simulink model "R1_double"  (R2014b)
settings: Solver=ode3  SolverMode=SingleTasking  StartTime=0.0  StopTime=Tsim  FixedStep=Ts  RelTol=1e-3
InitFcn:
  | configDoubleIntegrator
libraries: simulink x1
settings Model: CovMetricSettings=dwe  CovHtmlReporting=off  covSaveCumulativeToWorkspaceVar=off  CovSaveSingleToWorkspaceVar=off  CovExternalEMLEnable=on  CovSFcnEnable=on  Creator=mnade  LastModifiedBy=nina
settings DataIOCC: LimitDataPoints=off  SaveFormat=StructureWithTime
settings DebuggingCC: SolverPrmCheckMsg=none  FrameProcessingCompatibilityMsg=error  SFUnexpectedBacktrackingDiag=error  SFNoUnconditionalDefaultTransitionDiag=error
settings HardwareCC: ProdBitPerPointer=64  ProdLargestAtomicFloat=Float  ProdIntDivRoundTo=Zero  ProdEndianess=LittleEndian  ProdHWDeviceType=Specified
settings ModelReferenceCC: PropagateSignalLabelsOutOfModel=on
settings GRTTargetCC: TargetLangStandard=C99 (ISO)  GeneratePreprocessorConditionals=Use local settings

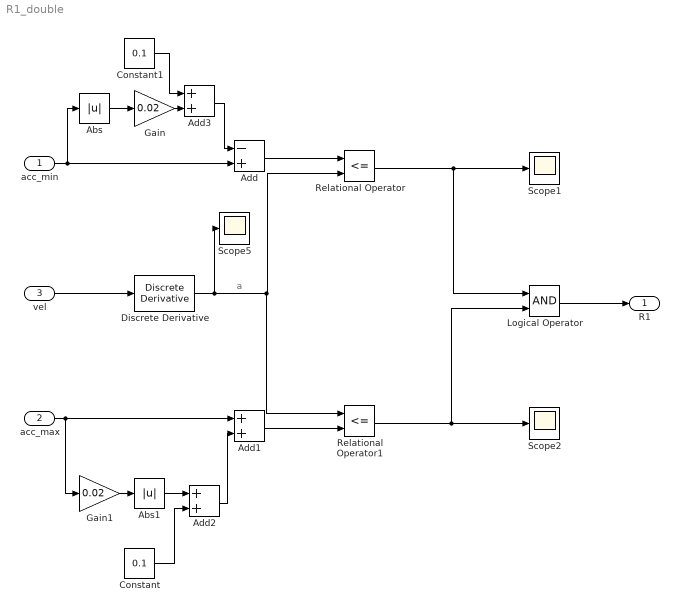
== system R1_double ==
  note: a
  acc_min : Inport
  acc_max : Inport  Port=2
  vel : Inport  Port=3
  Abs : Abs
  Abs1 : Abs
  Add : Sum  Inputs=-+
  Add1 : Sum
  Add2 : Sum
  Add3 : Sum
  Constant : Constant  Value=0.1
  Constant1 : Constant  Value=0.1
  Discrete Derivative : simulink/Discrete/Discrete Derivative  gainval=1.0  ICPrevScaledInput=0.0  InputProcessing=Inherited  OutMin=[]  OutMax=[]  OutDataType=fixdt(1, 16)  OutScaling=2^-10  DoSatur=off
  Gain : Gain  Gain=0.02
  Gain1 : Gain  Gain=0.02
  Logical Operator : Logic  AllPortsSameDT=off  OutDataTypeStr=boolean
  Relational Operator : RelationalOperator  Operator=<=  OutDataTypeStr=boolean
  Relational Operator1 : RelationalOperator  Operator=<=  OutDataTypeStr=boolean
  Scope1 : Scope
  Scope2 : Scope
  Scope5 : Scope
      settings: SaveName=ScopeData5
  R1 : Outport
  wires:
  vel/1 -> Discrete Derivative/1
  Discrete Derivative/1 -> Scope5/1, Relational Operator1/1, Relational Operator/2
  acc_min/1 -> Abs/1, Add/2
  acc_max/1 -> Gain1/1, Add1/1
  Relational Operator/1 -> Scope1/1, Logical Operator/1
  Logical Operator/1 -> R1/1
  Add/1 -> Relational Operator/1
  Add1/1 -> Relational Operator1/2
  Gain1/1 -> Abs1/1
  Gain/1 -> Add3/2
  Relational Operator1/1 -> Logical Operator/2, Scope2/1
  Abs/1 -> Gain/1
  Abs1/1 -> Add2/1
  Add2/1 -> Add1/2
  Add3/1 -> Add/1
  Constant1/1 -> Add3/1
  Constant/1 -> Add2/2
